simulink model "HW04_Demo"  (R2023b)
settings: Solver=VariableStepAuto  StartTime=0.0  StopTime=120  RelTol=1e-3
settings Model: Creator=ssjang  LastModifiedBy=YYlab_05
settings OptimizationCC: ReuseModelBlockBuffer=off

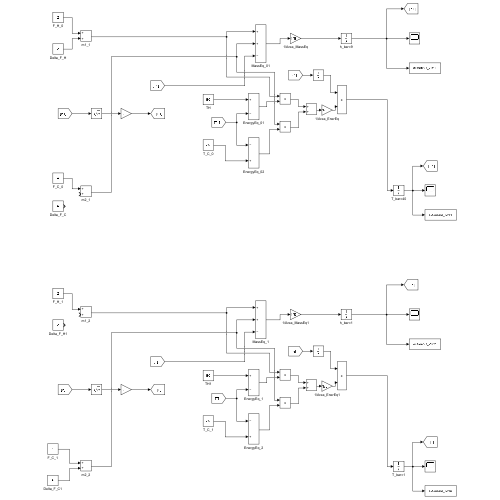
[thumbnail: Simulink's stored preview of the top-level diagram]
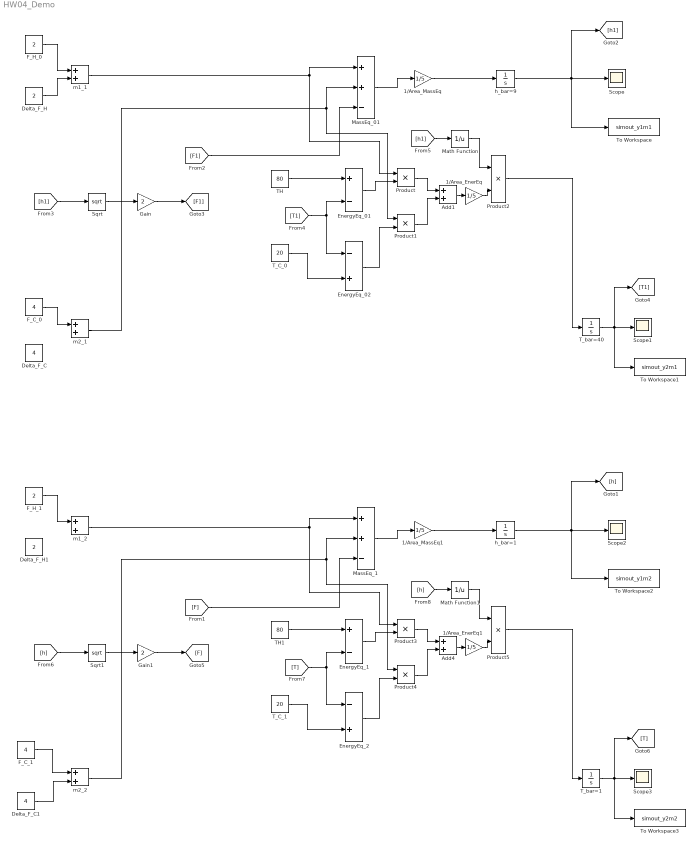
== system HW04_Demo ==
  1/Area_EnerEq : Gain  Gain=1/5
  1/Area_EnerEq1 : Gain  Gain=1/5
  1/Area_MassEq : Gain  Gain=1/5
  1/Area_MassEq1 : Gain  Gain=1/5
  Add1 : Sum
  Add4 : Sum
  Delta_F_C : Constant  Value=4
  Delta_F_C1 : Constant  Value=4
  Delta_F_H : Constant  Value=2
  Delta_F_H1 : Constant  Value=2
  EnergyEq_01 : Sum  Inputs=+-
  EnergyEq_02 : Sum  Inputs=-+
  EnergyEq_1 : Sum  Inputs=+-
  EnergyEq_2 : Sum  Inputs=-+
  F_C_0 : Constant  Value=4
  F_C_1 : Constant  Value=4
  F_H_0 : Constant  Value=2
  F_H_1 : Constant  Value=2
  Gain : Gain  Gain=2
  Gain1 : Gain  Gain=2
  MassEq_01 : Sum  Inputs=++-
  MassEq_1 : Sum  Inputs=++-
  Math Function : Math  Operator=reciprocal
  Math Function1 : Math  Operator=reciprocal
  Product{,1..5} (6 alike) : Product
  Scope{,1..3} (4 alike) : Scope
  Sqrt : Sqrt
  Sqrt1 : Sqrt
  TH : Constant  Value=80
  TH1 : Constant  Value=80
  T_C_0 : Constant  Value=20
  T_C_1 : Constant  Value=20
  T_bar=1 : Integrator  InitialCondition=40
  T_bar=40 : Integrator  InitialCondition=40
  To Workspace : ToWorkspace  VariableName=simout_y1m1  SaveFormat=Timeseries  SampleTime=-1
  To Workspace1 : ToWorkspace  VariableName=simout_y2m1  SaveFormat=Timeseries  SampleTime=-1
  To Workspace2 : ToWorkspace  VariableName=simout_y1m2  SaveFormat=Timeseries  SampleTime=-1
  To Workspace3 : ToWorkspace  VariableName=simout_y2m2  SaveFormat=Timeseries  SampleTime=-1
  h_bar=1 : Integrator  InitialCondition=9
  h_bar=9 : Integrator  InitialCondition=9
  m1_1 : Sum
  m1_2 : Sum
  m2_1 : Sum
  m2_2 : Sum
  wires:
  m2_1/1 -> MassEq_01/2, Product1/1
  [F1] -> MassEq_01/3
  MassEq_01/1 -> 1/Area_MassEq/1
  1/Area_MassEq/1 -> h_bar=9/1
  h_bar=9/1 -> [h1], To Workspace/1, Scope/1
  [h1] -> Sqrt/1
  Sqrt/1 -> Gain/1
  Gain/1 -> [F1]
  T_bar=40/1 -> [T1], To Workspace1/1, Scope1/1
  TH/1 -> EnergyEq_01/1
  [T1] -> EnergyEq_01/2, EnergyEq_02/1
  EnergyEq_01/1 -> Product/2
  Product/1 -> Add1/1
  T_C_0/1 -> EnergyEq_02/2
  EnergyEq_02/1 -> Product1/2
  Product1/1 -> Add1/2
  Add1/1 -> 1/Area_EnerEq/1
  1/Area_EnerEq/1 -> Product2/2
  Product2/1 -> T_bar=40/1
  [h1] -> Math Function/1
  Math Function/1 -> Product2/1
  m1_1/1 -> MassEq_01/1, Product/1
  Delta_F_H/1 -> m1_1/2
  F_H_0/1 -> m1_1/1
  F_C_0/1 -> m2_1/1
  m2_2/1 -> MassEq_1/2, Product4/1
  Delta_F_C1/1 -> m2_2/2
  [T] -> EnergyEq_1/2, EnergyEq_2/1
  F_C_1/1 -> m2_2/1
  Product3/1 -> Add4/1
  1/Area_EnerEq1/1 -> Product5/2
  F_H_1/1 -> m1_2/1
  TH1/1 -> EnergyEq_1/1
  T_C_1/1 -> EnergyEq_2/2
  1/Area_MassEq1/1 -> h_bar=1/1
  m1_2/1 -> MassEq_1/1, Product3/1
  Product5/1 -> T_bar=1/1
  [h] -> Sqrt1/1
  EnergyEq_1/1 -> Product3/2
  Product4/1 -> Add4/2
  [h] -> Math Function1/1
  Math Function1/1 -> Product5/1
  T_bar=1/1 -> [T], To Workspace3/1, Scope3/1
  EnergyEq_2/1 -> Product4/2
  h_bar=1/1 -> [h], To Workspace2/1, Scope2/1
  MassEq_1/1 -> 1/Area_MassEq1/1
  Gain1/1 -> [F]
  Add4/1 -> 1/Area_EnerEq1/1
  Sqrt1/1 -> Gain1/1
  [F] -> MassEq_1/3
